simulink model "warp_timer"  (Simulink 7.1)
settings: Solver=ode45  StartTime=0.0  StopTime=1000  RelTol=1e-3
undefined symbols (not defined in the file): gcbh, xlBlockLoadCallback, xlGetSimulinkPeriod
libraries: xbsIndex_r4 x450
(part 3 of 5)

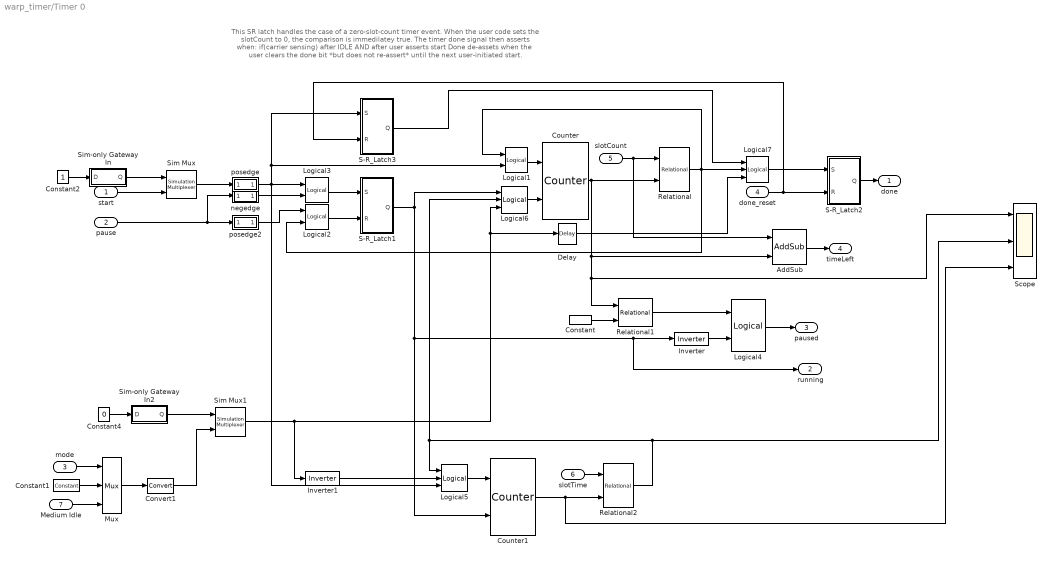
== system warp_timer/Timer 0 ==
  note: This SR latch handles the case of a zero-slot-count
      | timer event. When the user code sets the slotCount to 0,
      | the comparison is immedilatey true. The timer done
      | signal then asserts when:
      | if(carrier sensing) after IDLE AND
      | after user asserts start
      | Done de-assets when the user clears the done bit
      | *but does not re-assert* until the next user-initiated start.
  start : Inport  OutDataType=sfix(16)  OutScaling=2^0
  pause : Inport  Port=2  OutDataType=sfix(16)  OutScaling=2^0
  mode : Inport  Port=3  OutDataType=sfix(16)  OutScaling=2^0
  done_reset : Inport  Port=4  OutDataType=sfix(16)  OutScaling=2^0
  slotCount : Inport  Port=5  OutDataType=sfix(16)  OutScaling=2^0
  slotTime : Inport  Port=6  OutDataType=sfix(16)  OutScaling=2^0
  Medium Idle : Inport  Port=7  OutDataType=sfix(16)  OutScaling=2^0
  AddSub : xbsIndex_r4/AddSub  mode=Subtraction  use_carryin=off  use_carryout=off  en=off  latency=0  precision=User Defined  arith_type=Unsigned  n_bits=32  bin_pt=0  quantization=Truncate  overflow=Wrap  dbl_ovrd=off  use_behavioral_HDL=off  pipelined=off  use_rpm=on  hw_selection=Fabric  block_type=addsub
      settings: xl_area=[16 0 0 32 0 0 0]  block_version=8.2
  Constant : xbsIndex_r4/Constant  arith_type=Unsigned  const=0  n_bits=32  bin_pt=0  explicit_period=off  period=1  equ=P=C  opselect=C  inp2=PCIN>>17  opr=+  inp1=P  carry=CIN  dbl_ovrd=off  block_type=constant
      settings: block_version=10.1.2
  Constant1 : xbsIndex_r4/Constant  arith_type=Unsigned  const=1  n_bits=1  bin_pt=0  explicit_period=off  period=1  equ=P=C  opselect=C  inp2=PCIN>>17  opr=+  inp1=P  carry=CIN  dbl_ovrd=off  block_type=constant
      settings: block_version=8.2
  Constant2 : Constant  OutDataType=sfix(16)  OutScaling=2^0
  Constant4 : Constant  Value=0  OutDataType=sfix(16)  OutScaling=2^0
  Convert1 : xbsIndex_r4/Convert  arith_type=Boolean  n_bits=16  bin_pt=14  quantization=Truncate  overflow=Wrap  latency=0  dbl_ovrd=off  pipeline=off  block_type=convert
      settings: xl_area=[0 0 0 0 0 0 0]  block_version=8.2
  Counter : xbsIndex_r4/Counter  cnt_type=Free Running  cnt_to=Inf  operation=Up  start_count=0  cnt_by_val=1  arith_type=Unsigned  n_bits=32  bin_pt=0  load_pin=off  rst=on  en=on  explicit_period=on  period=1  dbl_ovrd=off  use_behavioral_HDL=off  use_rpm=off  implementation=Fabric  block_type=counter
      settings: xl_area=[17 32 0 32 0 0 0]  block_version=8.2
  Counter1 : xbsIndex_r4/Counter  cnt_type=Free Running  cnt_to=Inf  operation=Up  start_count=0  cnt_by_val=1  arith_type=Unsigned  n_bits=16  bin_pt=0  load_pin=off  rst=on  en=on  explicit_period=on  period=1  dbl_ovrd=off  use_behavioral_HDL=off  use_rpm=off  implementation=Fabric  block_type=counter
      settings: xl_area=[17 32 0 32 0 0 0]  block_version=8.2
  Delay : xbsIndex_r4/Delay  en=off  latency=1  dbl_ovrd=off  reg_retiming=off  block_type=delay
  Inverter : xbsIndex_r4/Inverter  en=off  latency=0  dbl_ovrd=off  block_type=inv
      settings: xl_area=[0 0 0 0 0 0 0]  block_version=10.1.2
  Inverter1 : xbsIndex_r4/Inverter  en=off  latency=0  dbl_ovrd=off  block_type=inv
      settings: xl_area=[0 0 0 0 0 0 0]  block_version=10.1.2
  Logical1 : xbsIndex_r4/Logical  logical_function=OR  inputs=2  en=off  latency=0  precision=Full  arith_type=Unsigned  n_bits=16  bin_pt=0  align_bp=on  dbl_ovrd=off  block_type=logical
      settings: xl_area=[1 0 0 1 0 0 0]  block_version=9.1.01
  Logical2 : xbsIndex_r4/Logical  logical_function=OR  inputs=2  en=off  latency=0  precision=Full  arith_type=Unsigned  n_bits=16  bin_pt=0  align_bp=on  dbl_ovrd=off  block_type=logical
      settings: xl_area=[1 0 0 1 0 0 0]  block_version=9.1.01
  Logical3 : xbsIndex_r4/Logical  logical_function=OR  inputs=2  en=off  latency=0  precision=Full  arith_type=Unsigned  n_bits=16  bin_pt=0  align_bp=on  dbl_ovrd=off  block_type=logical
      settings: xl_area=[1 0 0 1 0 0 0]  block_version=9.1.01
  Logical4 : xbsIndex_r4/Logical  logical_function=AND  inputs=2  en=off  latency=0  precision=Full  arith_type=Unsigned  n_bits=16  bin_pt=0  align_bp=on  dbl_ovrd=off  block_type=logical
      settings: xl_area=[1 0 0 1 0 0 0]  block_version=10.1.2
  Logical5 : xbsIndex_r4/Logical  logical_function=OR  inputs=3  en=off  latency=0  precision=Full  arith_type=Unsigned  n_bits=16  bin_pt=0  align_bp=on  dbl_ovrd=off  block_type=logical
      settings: xl_area=[1 0 0 1 0 0 0]  block_version=8.2
  Logical6 : xbsIndex_r4/Logical  logical_function=AND  inputs=3  en=off  latency=0  precision=Full  arith_type=Unsigned  n_bits=16  bin_pt=0  align_bp=on  dbl_ovrd=off  block_type=logical
      settings: xl_area=[1 0 0 1 0 0 0]  block_version=8.2
  Logical7 : xbsIndex_r4/Logical  logical_function=AND  inputs=3  en=off  latency=0  precision=Full  arith_type=Unsigned  n_bits=16  bin_pt=0  align_bp=on  dbl_ovrd=off  block_type=logical
      settings: xl_area=[1 0 0 1 0 0 0]  block_version=9.1.01
  Mux : xbsIndex_r4/Mux  inputs=2  en=off  latency=0  precision=Full  arith_type=Unsigned  n_bits=16  bin_pt=14  quantization=Truncate  overflow=Wrap  dbl_ovrd=off  block_type=mux
      settings: xl_area=[1 0 0 1 0 0 0]  block_version=8.2
  Relational : xbsIndex_r4/Relational  mode=a<=b  en=off  latency=0  dbl_ovrd=off  block_type=relational
      settings: xl_area=[8 0 0 16 0 0 0]  block_version=8.2
  Relational1 : xbsIndex_r4/Relational  mode=a>b  en=off  latency=0  dbl_ovrd=off  block_type=relational
      settings: xl_area=[16 1 0 32 0 0 0]  block_version=10.1.2
  Relational2 : xbsIndex_r4/Relational  mode=a<=b  en=off  latency=0  dbl_ovrd=off  block_type=relational
      settings: xl_area=[8 0 0 16 0 0 0]  block_version=8.2
  S-R_Latch1 : Subsystem
  S-R_Latch2 : Subsystem
  S-R_Latch3 : Subsystem
  Scope : Scope  NumInputPorts=3
      settings: YMin=-5~-5~-5  YMax=5~5~5
  Sim Mux : xbsIndex_r4/Simulation Multiplexer  sim_sel=1  hw_sel=2  block_type=simmux
      settings: infoedit="Distinguish input subsystems as \"simulation only\" and \"generation only\".  The input specified For Simulation will be used during Simulink simulation.  The input specified For Generation will be used during code generation.  This block will typically be used on the output of a HW Co-Simulation, Black Box, or ModelSim subsystem.<P><P>Hardware Notes: This block costs nothing."  block_version=10.1.3
  Sim Mux1 : xbsIndex_r4/Simulation Multiplexer  sim_sel=1  hw_sel=2  block_type=simmux
      settings: infoedit="Distinguish input subsystems as \"simulation only\" and \"generation only\".  The input specified For Simulation will be used during Simulink simulation.  The input specified For Generation will be used during code generation.  This block will typically be used on the output of a HW Co-Simulation, Black Box, or ModelSim subsystem.<P><P>Hardware Notes: This block costs nothing."  block_version=10.1.3
  Sim-only Gateway In : Subsystem
  Sim-only Gateway In2 : Subsystem
  negedge : Subsystem
  posedge : Subsystem
  posedge2 : Subsystem
  done : Outport  OutDataType=sfix(16)  OutScaling=2^0
  running : Outport  Port=2  OutDataType=sfix(16)  OutScaling=2^0
  paused : Outport  Port=3  OutDataType=sfix(16)  OutScaling=2^0
  timeLeft : Outport  Port=4  OutDataType=sfix(16)  OutScaling=2^0
  wires:
  mode/1 -> Mux/1
  Constant1/1 -> Mux/2
  Medium Idle/1 -> Mux/3
  Mux/1 -> Convert1/1
  Logical4/1 -> paused/1
  start/1 -> Sim Mux/2
  Sim Mux/1 -> posedge/1(In)
  AddSub/1 -> timeLeft/1
  Constant/1 -> Relational1/2
  Relational1/1 -> Logical4/1
  Inverter/1 -> Logical4/2
  S-R_Latch1/1(Q) -> Counter1/2, Inverter/1, running/1, Logical6/1
  slotCount/1 -> AddSub/1, Relational/1
  Counter/1 -> Relational/2, AddSub/2, Relational1/1, Scope/1
  Logical1/1 -> Counter/1
  S-R_Latch2/1(Q) -> done/1
  Relational/1 -> Logical2/2, Logical1/1, Logical7/2
  done_reset/1 -> S-R_Latch2/2(R), S-R_Latch3/2(R)
  posedge/1(Out) -> Logical3/1, Logical5/3, Logical1/2, S-R_Latch3/1(S)
  Logical3/1 -> S-R_Latch1/1(S)
  negedge/1(Out) -> Logical3/2
  pause/1 -> posedge2/1(In), negedge/1(In)
  Sim-only Gateway In/1(Q) -> Sim Mux/1
  slotTime/1 -> Relational2/1
  Counter1/1 -> Relational2/2, Scope/3
  Logical5/1 -> Counter1/1
  Relational2/1 -> Logical5/1, Logical6/2, Scope/2
  Inverter1/1 -> Logical5/2
  Logical6/1 -> Counter/2
  Convert1/1 -> Sim Mux1/2
  Sim Mux1/1 -> Inverter1/1, Logical6/3, Delay/1
  Constant2/1 -> Sim-only Gateway In/1(D)
  posedge2/1(Out) -> Logical2/1
  Logical2/1 -> S-R_Latch1/2(R)
  Constant4/1 -> Sim-only Gateway In2/1(D)
  Sim-only Gateway In2/1(Q) -> Sim Mux1/1
  Logical7/1 -> S-R_Latch2/1(S)
  S-R_Latch3/1(Q) -> Logical7/1
  Delay/1 -> Logical7/3

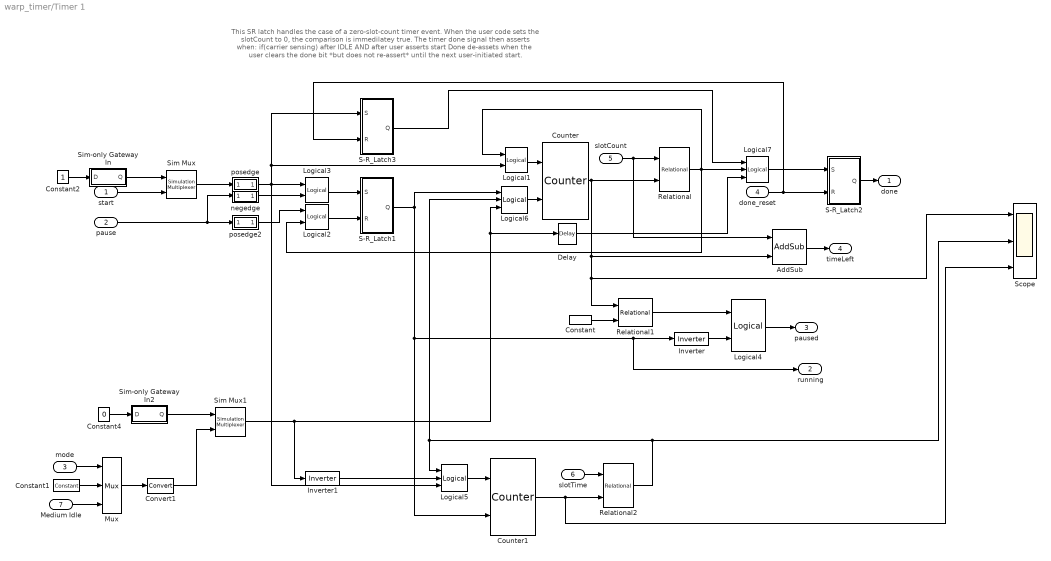
== system warp_timer/Timer 1 ==
  note: This SR latch handles the case of a zero-slot-count
      | timer event. When the user code sets the slotCount to 0,
      | the comparison is immedilatey true. The timer done
      | signal then asserts when:
      | if(carrier sensing) after IDLE AND
      | after user asserts start
      | Done de-assets when the user clears the done bit
      | *but does not re-assert* until the next user-initiated start.
  start : Inport  OutDataType=sfix(16)  OutScaling=2^0
  pause : Inport  Port=2  OutDataType=sfix(16)  OutScaling=2^0
  mode : Inport  Port=3  OutDataType=sfix(16)  OutScaling=2^0
  done_reset : Inport  Port=4  OutDataType=sfix(16)  OutScaling=2^0
  slotCount : Inport  Port=5  OutDataType=sfix(16)  OutScaling=2^0
  slotTime : Inport  Port=6  OutDataType=sfix(16)  OutScaling=2^0
  Medium Idle : Inport  Port=7  OutDataType=sfix(16)  OutScaling=2^0
  AddSub : xbsIndex_r4/AddSub  mode=Subtraction  use_carryin=off  use_carryout=off  en=off  latency=0  precision=User Defined  arith_type=Unsigned  n_bits=32  bin_pt=0  quantization=Truncate  overflow=Wrap  dbl_ovrd=off  use_behavioral_HDL=off  pipelined=off  use_rpm=on  hw_selection=Fabric  block_type=addsub
      settings: xl_area=[16 0 0 32 0 0 0]  block_version=8.2
  Constant : xbsIndex_r4/Constant  arith_type=Unsigned  const=0  n_bits=32  bin_pt=0  explicit_period=off  period=1  equ=P=C  opselect=C  inp2=PCIN>>17  opr=+  inp1=P  carry=CIN  dbl_ovrd=off  block_type=constant
      settings: block_version=10.1.2
  Constant1 : xbsIndex_r4/Constant  arith_type=Unsigned  const=1  n_bits=1  bin_pt=0  explicit_period=off  period=1  equ=P=C  opselect=C  inp2=PCIN>>17  opr=+  inp1=P  carry=CIN  dbl_ovrd=off  block_type=constant
      settings: block_version=8.2
  Constant2 : Constant  OutDataType=sfix(16)  OutScaling=2^0
  Constant4 : Constant  Value=0  OutDataType=sfix(16)  OutScaling=2^0
  Convert1 : xbsIndex_r4/Convert  arith_type=Boolean  n_bits=16  bin_pt=14  quantization=Truncate  overflow=Wrap  latency=0  dbl_ovrd=off  pipeline=off  block_type=convert
      settings: xl_area=[0 0 0 0 0 0 0]  block_version=8.2
  Counter : xbsIndex_r4/Counter  cnt_type=Free Running  cnt_to=Inf  operation=Up  start_count=0  cnt_by_val=1  arith_type=Unsigned  n_bits=32  bin_pt=0  load_pin=off  rst=on  en=on  explicit_period=on  period=1  dbl_ovrd=off  use_behavioral_HDL=off  use_rpm=off  implementation=Fabric  block_type=counter
      settings: xl_area=[17 32 0 32 0 0 0]  block_version=8.2
  Counter1 : xbsIndex_r4/Counter  cnt_type=Free Running  cnt_to=Inf  operation=Up  start_count=0  cnt_by_val=1  arith_type=Unsigned  n_bits=16  bin_pt=0  load_pin=off  rst=on  en=on  explicit_period=on  period=1  dbl_ovrd=off  use_behavioral_HDL=off  use_rpm=off  implementation=Fabric  block_type=counter
      settings: xl_area=[17 32 0 32 0 0 0]  block_version=8.2
  Delay : xbsIndex_r4/Delay  en=off  latency=1  dbl_ovrd=off  reg_retiming=off  block_type=delay
  Inverter : xbsIndex_r4/Inverter  en=off  latency=0  dbl_ovrd=off  block_type=inv
      settings: xl_area=[0 0 0 0 0 0 0]  block_version=10.1.2
  Inverter1 : xbsIndex_r4/Inverter  en=off  latency=0  dbl_ovrd=off  block_type=inv
      settings: xl_area=[0 0 0 0 0 0 0]  block_version=10.1.2
  Logical1 : xbsIndex_r4/Logical  logical_function=OR  inputs=2  en=off  latency=0  precision=Full  arith_type=Unsigned  n_bits=16  bin_pt=0  align_bp=on  dbl_ovrd=off  block_type=logical
      settings: xl_area=[1 0 0 1 0 0 0]  block_version=9.1.01
  Logical2 : xbsIndex_r4/Logical  logical_function=OR  inputs=2  en=off  latency=0  precision=Full  arith_type=Unsigned  n_bits=16  bin_pt=0  align_bp=on  dbl_ovrd=off  block_type=logical
      settings: xl_area=[1 0 0 1 0 0 0]  block_version=9.1.01
  Logical3 : xbsIndex_r4/Logical  logical_function=OR  inputs=2  en=off  latency=0  precision=Full  arith_type=Unsigned  n_bits=16  bin_pt=0  align_bp=on  dbl_ovrd=off  block_type=logical
      settings: xl_area=[1 0 0 1 0 0 0]  block_version=9.1.01
  Logical4 : xbsIndex_r4/Logical  logical_function=AND  inputs=2  en=off  latency=0  precision=Full  arith_type=Unsigned  n_bits=16  bin_pt=0  align_bp=on  dbl_ovrd=off  block_type=logical
      settings: xl_area=[1 0 0 1 0 0 0]  block_version=10.1.2
  Logical5 : xbsIndex_r4/Logical  logical_function=OR  inputs=3  en=off  latency=0  precision=Full  arith_type=Unsigned  n_bits=16  bin_pt=0  align_bp=on  dbl_ovrd=off  block_type=logical
      settings: xl_area=[1 0 0 1 0 0 0]  block_version=8.2
  Logical6 : xbsIndex_r4/Logical  logical_function=AND  inputs=3  en=off  latency=0  precision=Full  arith_type=Unsigned  n_bits=16  bin_pt=0  align_bp=on  dbl_ovrd=off  block_type=logical
      settings: xl_area=[1 0 0 1 0 0 0]  block_version=8.2
  Logical7 : xbsIndex_r4/Logical  logical_function=AND  inputs=3  en=off  latency=0  precision=Full  arith_type=Unsigned  n_bits=16  bin_pt=0  align_bp=on  dbl_ovrd=off  block_type=logical
      settings: xl_area=[1 0 0 1 0 0 0]  block_version=9.1.01
  Mux : xbsIndex_r4/Mux  inputs=2  en=off  latency=0  precision=Full  arith_type=Unsigned  n_bits=16  bin_pt=14  quantization=Truncate  overflow=Wrap  dbl_ovrd=off  block_type=mux
      settings: xl_area=[1 0 0 1 0 0 0]  block_version=8.2
  Relational : xbsIndex_r4/Relational  mode=a<=b  en=off  latency=0  dbl_ovrd=off  block_type=relational
      settings: xl_area=[8 0 0 16 0 0 0]  block_version=8.2
  Relational1 : xbsIndex_r4/Relational  mode=a>b  en=off  latency=0  dbl_ovrd=off  block_type=relational
      settings: xl_area=[16 1 0 32 0 0 0]  block_version=10.1.2
  Relational2 : xbsIndex_r4/Relational  mode=a<=b  en=off  latency=0  dbl_ovrd=off  block_type=relational
      settings: xl_area=[8 0 0 16 0 0 0]  block_version=8.2
  S-R_Latch1 : Subsystem
  S-R_Latch2 : Subsystem
  S-R_Latch3 : Subsystem
  Scope : Scope  NumInputPorts=3
      settings: YMin=-5~-5~-5  YMax=5~5~5
  Sim Mux : xbsIndex_r4/Simulation Multiplexer  sim_sel=1  hw_sel=2  block_type=simmux
      settings: infoedit="Distinguish input subsystems as \"simulation only\" and \"generation only\".  The input specified For Simulation will be used during Simulink simulation.  The input specified For Generation will be used during code generation.  This block will typically be used on the output of a HW Co-Simulation, Black Box, or ModelSim subsystem.<P><P>Hardware Notes: This block costs nothing."  block_version=10.1.3
  Sim Mux1 : xbsIndex_r4/Simulation Multiplexer  sim_sel=1  hw_sel=2  block_type=simmux
      settings: infoedit="Distinguish input subsystems as \"simulation only\" and \"generation only\".  The input specified For Simulation will be used during Simulink simulation.  The input specified For Generation will be used during code generation.  This block will typically be used on the output of a HW Co-Simulation, Black Box, or ModelSim subsystem.<P><P>Hardware Notes: This block costs nothing."  block_version=10.1.3
  Sim-only Gateway In : Subsystem
  Sim-only Gateway In2 : Subsystem
  negedge : Subsystem
  posedge : Subsystem
  posedge2 : Subsystem
  done : Outport  OutDataType=sfix(16)  OutScaling=2^0
  running : Outport  Port=2  OutDataType=sfix(16)  OutScaling=2^0
  paused : Outport  Port=3  OutDataType=sfix(16)  OutScaling=2^0
  timeLeft : Outport  Port=4  OutDataType=sfix(16)  OutScaling=2^0
  wires:
  Delay/1 -> Logical7/3
  S-R_Latch3/1(Q) -> Logical7/1
  Logical7/1 -> S-R_Latch2/1(S)
  Sim-only Gateway In2/1(Q) -> Sim Mux1/1
  Constant4/1 -> Sim-only Gateway In2/1(D)
  Logical2/1 -> S-R_Latch1/2(R)
  posedge2/1(Out) -> Logical2/1
  Constant2/1 -> Sim-only Gateway In/1(D)
  Sim Mux1/1 -> Delay/1, Logical6/3, Inverter1/1
  Convert1/1 -> Sim Mux1/2
  Logical6/1 -> Counter/2
  Inverter1/1 -> Logical5/2
  Relational2/1 -> Scope/2, Logical6/2, Logical5/1
  Logical5/1 -> Counter1/1
  Counter1/1 -> Scope/3, Relational2/2
  slotTime/1 -> Relational2/1
  Sim-only Gateway In/1(Q) -> Sim Mux/1
  pause/1 -> negedge/1(In), posedge2/1(In)
  negedge/1(Out) -> Logical3/2
  Logical3/1 -> S-R_Latch1/1(S)
  posedge/1(Out) -> S-R_Latch3/1(S), Logical1/2, Logical5/3, Logical3/1
  done_reset/1 -> S-R_Latch3/2(R), S-R_Latch2/2(R)
  Relational/1 -> Logical7/2, Logical1/1, Logical2/2
  S-R_Latch2/1(Q) -> done/1
  Logical1/1 -> Counter/1
  Counter/1 -> Scope/1, Relational1/1, AddSub/2, Relational/2
  slotCount/1 -> Relational/1, AddSub/1
  S-R_Latch1/1(Q) -> Logical6/1, running/1, Inverter/1, Counter1/2
  Inverter/1 -> Logical4/2
  Relational1/1 -> Logical4/1
  Constant/1 -> Relational1/2
  AddSub/1 -> timeLeft/1
  Sim Mux/1 -> posedge/1(In)
  start/1 -> Sim Mux/2
  Logical4/1 -> paused/1
  Mux/1 -> Convert1/1
  Medium Idle/1 -> Mux/3
  Constant1/1 -> Mux/2
  mode/1 -> Mux/1

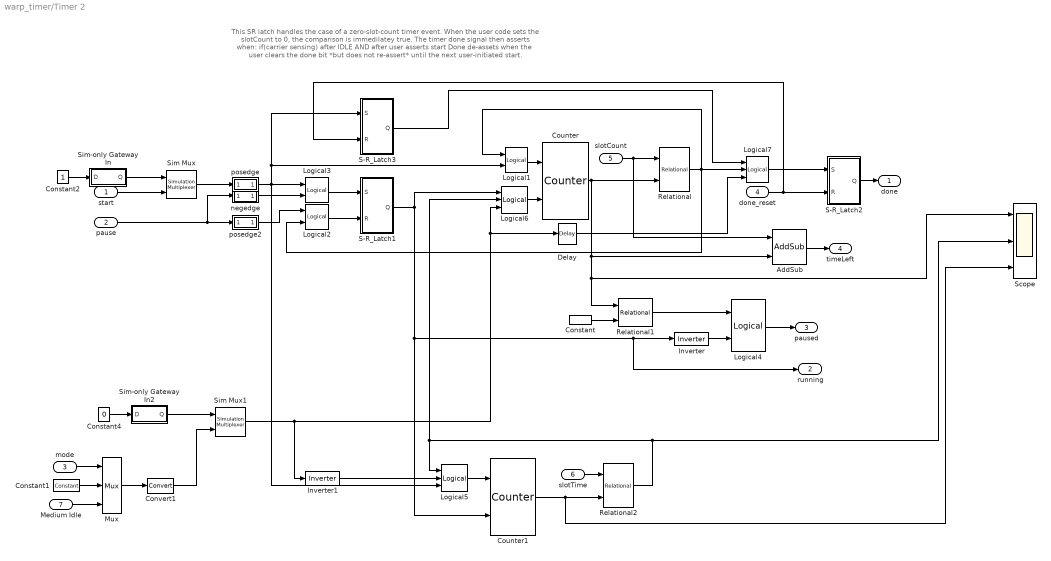
== system warp_timer/Timer 2 ==
  note: This SR latch handles the case of a zero-slot-count
      | timer event. When the user code sets the slotCount to 0,
      | the comparison is immedilatey true. The timer done
      | signal then asserts when:
      | if(carrier sensing) after IDLE AND
      | after user asserts start
      | Done de-assets when the user clears the done bit
      | *but does not re-assert* until the next user-initiated start.
  start : Inport  OutDataType=sfix(16)  OutScaling=2^0
  pause : Inport  Port=2  OutDataType=sfix(16)  OutScaling=2^0
  mode : Inport  Port=3  OutDataType=sfix(16)  OutScaling=2^0
  done_reset : Inport  Port=4  OutDataType=sfix(16)  OutScaling=2^0
  slotCount : Inport  Port=5  OutDataType=sfix(16)  OutScaling=2^0
  slotTime : Inport  Port=6  OutDataType=sfix(16)  OutScaling=2^0
  Medium Idle : Inport  Port=7  OutDataType=sfix(16)  OutScaling=2^0
  AddSub : xbsIndex_r4/AddSub  mode=Subtraction  use_carryin=off  use_carryout=off  en=off  latency=0  precision=User Defined  arith_type=Unsigned  n_bits=32  bin_pt=0  quantization=Truncate  overflow=Wrap  dbl_ovrd=off  use_behavioral_HDL=off  pipelined=off  use_rpm=on  hw_selection=Fabric  block_type=addsub
      settings: xl_area=[16 0 0 32 0 0 0]  block_version=8.2
  Constant : xbsIndex_r4/Constant  arith_type=Unsigned  const=0  n_bits=32  bin_pt=0  explicit_period=off  period=1  equ=P=C  opselect=C  inp2=PCIN>>17  opr=+  inp1=P  carry=CIN  dbl_ovrd=off  block_type=constant
      settings: block_version=10.1.2
  Constant1 : xbsIndex_r4/Constant  arith_type=Unsigned  const=1  n_bits=1  bin_pt=0  explicit_period=off  period=1  equ=P=C  opselect=C  inp2=PCIN>>17  opr=+  inp1=P  carry=CIN  dbl_ovrd=off  block_type=constant
      settings: block_version=8.2
  Constant2 : Constant  OutDataType=sfix(16)  OutScaling=2^0
  Constant4 : Constant  Value=0  OutDataType=sfix(16)  OutScaling=2^0
  Convert1 : xbsIndex_r4/Convert  arith_type=Boolean  n_bits=16  bin_pt=14  quantization=Truncate  overflow=Wrap  latency=0  dbl_ovrd=off  pipeline=off  block_type=convert
      settings: xl_area=[0 0 0 0 0 0 0]  block_version=8.2
  Counter : xbsIndex_r4/Counter  cnt_type=Free Running  cnt_to=Inf  operation=Up  start_count=0  cnt_by_val=1  arith_type=Unsigned  n_bits=32  bin_pt=0  load_pin=off  rst=on  en=on  explicit_period=on  period=1  dbl_ovrd=off  use_behavioral_HDL=off  use_rpm=off  implementation=Fabric  block_type=counter
      settings: xl_area=[17 32 0 32 0 0 0]  block_version=8.2
  Counter1 : xbsIndex_r4/Counter  cnt_type=Free Running  cnt_to=Inf  operation=Up  start_count=0  cnt_by_val=1  arith_type=Unsigned  n_bits=16  bin_pt=0  load_pin=off  rst=on  en=on  explicit_period=on  period=1  dbl_ovrd=off  use_behavioral_HDL=off  use_rpm=off  implementation=Fabric  block_type=counter
      settings: xl_area=[17 32 0 32 0 0 0]  block_version=8.2
  Delay : xbsIndex_r4/Delay  en=off  latency=1  dbl_ovrd=off  reg_retiming=off  block_type=delay
  Inverter : xbsIndex_r4/Inverter  en=off  latency=0  dbl_ovrd=off  block_type=inv
      settings: xl_area=[0 0 0 0 0 0 0]  block_version=10.1.2
  Inverter1 : xbsIndex_r4/Inverter  en=off  latency=0  dbl_ovrd=off  block_type=inv
      settings: xl_area=[0 0 0 0 0 0 0]  block_version=10.1.2
  Logical1 : xbsIndex_r4/Logical  logical_function=OR  inputs=2  en=off  latency=0  precision=Full  arith_type=Unsigned  n_bits=16  bin_pt=0  align_bp=on  dbl_ovrd=off  block_type=logical
      settings: xl_area=[1 0 0 1 0 0 0]  block_version=9.1.01
  Logical2 : xbsIndex_r4/Logical  logical_function=OR  inputs=2  en=off  latency=0  precision=Full  arith_type=Unsigned  n_bits=16  bin_pt=0  align_bp=on  dbl_ovrd=off  block_type=logical
      settings: xl_area=[1 0 0 1 0 0 0]  block_version=9.1.01
  Logical3 : xbsIndex_r4/Logical  logical_function=OR  inputs=2  en=off  latency=0  precision=Full  arith_type=Unsigned  n_bits=16  bin_pt=0  align_bp=on  dbl_ovrd=off  block_type=logical
      settings: xl_area=[1 0 0 1 0 0 0]  block_version=9.1.01
  Logical4 : xbsIndex_r4/Logical  logical_function=AND  inputs=2  en=off  latency=0  precision=Full  arith_type=Unsigned  n_bits=16  bin_pt=0  align_bp=on  dbl_ovrd=off  block_type=logical
      settings: xl_area=[1 0 0 1 0 0 0]  block_version=10.1.2
  Logical5 : xbsIndex_r4/Logical  logical_function=OR  inputs=3  en=off  latency=0  precision=Full  arith_type=Unsigned  n_bits=16  bin_pt=0  align_bp=on  dbl_ovrd=off  block_type=logical
      settings: xl_area=[1 0 0 1 0 0 0]  block_version=8.2
  Logical6 : xbsIndex_r4/Logical  logical_function=AND  inputs=3  en=off  latency=0  precision=Full  arith_type=Unsigned  n_bits=16  bin_pt=0  align_bp=on  dbl_ovrd=off  block_type=logical
      settings: xl_area=[1 0 0 1 0 0 0]  block_version=8.2
  Logical7 : xbsIndex_r4/Logical  logical_function=AND  inputs=3  en=off  latency=0  precision=Full  arith_type=Unsigned  n_bits=16  bin_pt=0  align_bp=on  dbl_ovrd=off  block_type=logical
      settings: xl_area=[1 0 0 1 0 0 0]  block_version=9.1.01
  Mux : xbsIndex_r4/Mux  inputs=2  en=off  latency=0  precision=Full  arith_type=Unsigned  n_bits=16  bin_pt=14  quantization=Truncate  overflow=Wrap  dbl_ovrd=off  block_type=mux
      settings: xl_area=[1 0 0 1 0 0 0]  block_version=8.2
  Relational : xbsIndex_r4/Relational  mode=a<=b  en=off  latency=0  dbl_ovrd=off  block_type=relational
      settings: xl_area=[8 0 0 16 0 0 0]  block_version=8.2
  Relational1 : xbsIndex_r4/Relational  mode=a>b  en=off  latency=0  dbl_ovrd=off  block_type=relational
      settings: xl_area=[16 1 0 32 0 0 0]  block_version=10.1.2
  Relational2 : xbsIndex_r4/Relational  mode=a<=b  en=off  latency=0  dbl_ovrd=off  block_type=relational
      settings: xl_area=[8 0 0 16 0 0 0]  block_version=8.2
  S-R_Latch1 : Subsystem
  S-R_Latch2 : Subsystem
  S-R_Latch3 : Subsystem
  Scope : Scope  NumInputPorts=3
      settings: YMin=-5~-5~-5  YMax=5~5~5
  Sim Mux : xbsIndex_r4/Simulation Multiplexer  sim_sel=1  hw_sel=2  block_type=simmux
      settings: infoedit="Distinguish input subsystems as \"simulation only\" and \"generation only\".  The input specified For Simulation will be used during Simulink simulation.  The input specified For Generation will be used during code generation.  This block will typically be used on the output of a HW Co-Simulation, Black Box, or ModelSim subsystem.<P><P>Hardware Notes: This block costs nothing."  block_version=10.1.3
  Sim Mux1 : xbsIndex_r4/Simulation Multiplexer  sim_sel=1  hw_sel=2  block_type=simmux
      settings: infoedit="Distinguish input subsystems as \"simulation only\" and \"generation only\".  The input specified For Simulation will be used during Simulink simulation.  The input specified For Generation will be used during code generation.  This block will typically be used on the output of a HW Co-Simulation, Black Box, or ModelSim subsystem.<P><P>Hardware Notes: This block costs nothing."  block_version=10.1.3
  Sim-only Gateway In : Subsystem
  Sim-only Gateway In2 : Subsystem
  negedge : Subsystem
  posedge : Subsystem
  posedge2 : Subsystem
  done : Outport  OutDataType=sfix(16)  OutScaling=2^0
  running : Outport  Port=2  OutDataType=sfix(16)  OutScaling=2^0
  paused : Outport  Port=3  OutDataType=sfix(16)  OutScaling=2^0
  timeLeft : Outport  Port=4  OutDataType=sfix(16)  OutScaling=2^0
  wires:
  mode/1 -> Mux/1
  Constant1/1 -> Mux/2
  Medium Idle/1 -> Mux/3
  Mux/1 -> Convert1/1
  Logical4/1 -> paused/1
  start/1 -> Sim Mux/2
  Sim Mux/1 -> posedge/1(In)
  AddSub/1 -> timeLeft/1
  Constant/1 -> Relational1/2
  Relational1/1 -> Logical4/1
  Inverter/1 -> Logical4/2
  S-R_Latch1/1(Q) -> Counter1/2, Inverter/1, running/1, Logical6/1
  slotCount/1 -> AddSub/1, Relational/1
  Counter/1 -> Relational/2, AddSub/2, Relational1/1, Scope/1
  Logical1/1 -> Counter/1
  S-R_Latch2/1(Q) -> done/1
  Relational/1 -> Logical2/2, Logical1/1, Logical7/2
  done_reset/1 -> S-R_Latch2/2(R), S-R_Latch3/2(R)
  posedge/1(Out) -> Logical3/1, Logical5/3, Logical1/2, S-R_Latch3/1(S)
  Logical3/1 -> S-R_Latch1/1(S)
  negedge/1(Out) -> Logical3/2
  pause/1 -> posedge2/1(In), negedge/1(In)
  Sim-only Gateway In/1(Q) -> Sim Mux/1
  slotTime/1 -> Relational2/1
  Counter1/1 -> Relational2/2, Scope/3
  Logical5/1 -> Counter1/1
  Relational2/1 -> Logical5/1, Logical6/2, Scope/2
  Inverter1/1 -> Logical5/2
  Logical6/1 -> Counter/2
  Convert1/1 -> Sim Mux1/2
  Sim Mux1/1 -> Inverter1/1, Logical6/3, Delay/1
  Constant2/1 -> Sim-only Gateway In/1(D)
  posedge2/1(Out) -> Logical2/1
  Logical2/1 -> S-R_Latch1/2(R)
  Constant4/1 -> Sim-only Gateway In2/1(D)
  Sim-only Gateway In2/1(Q) -> Sim Mux1/1
  Logical7/1 -> S-R_Latch2/1(S)
  S-R_Latch3/1(Q) -> Logical7/1
  Delay/1 -> Logical7/3

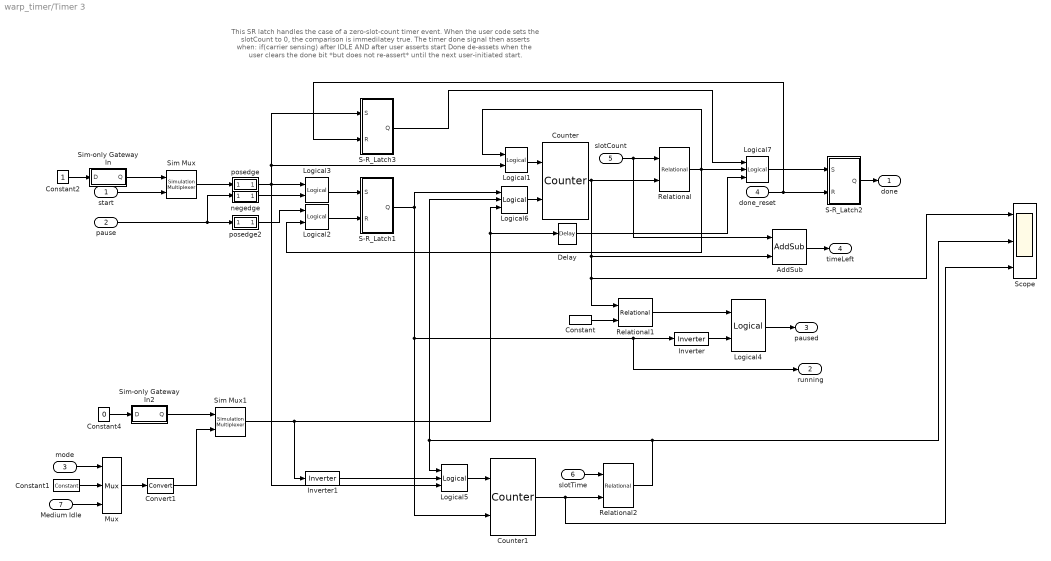
== system warp_timer/Timer 3 ==
  note: This SR latch handles the case of a zero-slot-count
      | timer event. When the user code sets the slotCount to 0,
      | the comparison is immedilatey true. The timer done
      | signal then asserts when:
      | if(carrier sensing) after IDLE AND
      | after user asserts start
      | Done de-assets when the user clears the done bit
      | *but does not re-assert* until the next user-initiated start.
  start : Inport  OutDataType=sfix(16)  OutScaling=2^0
  pause : Inport  Port=2  OutDataType=sfix(16)  OutScaling=2^0
  mode : Inport  Port=3  OutDataType=sfix(16)  OutScaling=2^0
  done_reset : Inport  Port=4  OutDataType=sfix(16)  OutScaling=2^0
  slotCount : Inport  Port=5  OutDataType=sfix(16)  OutScaling=2^0
  slotTime : Inport  Port=6  OutDataType=sfix(16)  OutScaling=2^0
  Medium Idle : Inport  Port=7  OutDataType=sfix(16)  OutScaling=2^0
  AddSub : xbsIndex_r4/AddSub  mode=Subtraction  use_carryin=off  use_carryout=off  en=off  latency=0  precision=User Defined  arith_type=Unsigned  n_bits=32  bin_pt=0  quantization=Truncate  overflow=Wrap  dbl_ovrd=off  use_behavioral_HDL=off  pipelined=off  use_rpm=on  hw_selection=Fabric  block_type=addsub
      settings: xl_area=[16 0 0 32 0 0 0]  block_version=8.2
  Constant : xbsIndex_r4/Constant  arith_type=Unsigned  const=0  n_bits=32  bin_pt=0  explicit_period=off  period=1  equ=P=C  opselect=C  inp2=PCIN>>17  opr=+  inp1=P  carry=CIN  dbl_ovrd=off  block_type=constant
      settings: block_version=10.1.2
  Constant1 : xbsIndex_r4/Constant  arith_type=Unsigned  const=1  n_bits=1  bin_pt=0  explicit_period=off  period=1  equ=P=C  opselect=C  inp2=PCIN>>17  opr=+  inp1=P  carry=CIN  dbl_ovrd=off  block_type=constant
      settings: block_version=8.2
  Constant2 : Constant  OutDataType=sfix(16)  OutScaling=2^0
  Constant4 : Constant  Value=0  OutDataType=sfix(16)  OutScaling=2^0
  Convert1 : xbsIndex_r4/Convert  arith_type=Boolean  n_bits=16  bin_pt=14  quantization=Truncate  overflow=Wrap  latency=0  dbl_ovrd=off  pipeline=off  block_type=convert
      settings: xl_area=[0 0 0 0 0 0 0]  block_version=8.2
  Counter : xbsIndex_r4/Counter  cnt_type=Free Running  cnt_to=Inf  operation=Up  start_count=0  cnt_by_val=1  arith_type=Unsigned  n_bits=32  bin_pt=0  load_pin=off  rst=on  en=on  explicit_period=on  period=1  dbl_ovrd=off  use_behavioral_HDL=off  use_rpm=off  implementation=Fabric  block_type=counter
      settings: xl_area=[17 32 0 32 0 0 0]  block_version=8.2
  Counter1 : xbsIndex_r4/Counter  cnt_type=Free Running  cnt_to=Inf  operation=Up  start_count=0  cnt_by_val=1  arith_type=Unsigned  n_bits=16  bin_pt=0  load_pin=off  rst=on  en=on  explicit_period=on  period=1  dbl_ovrd=off  use_behavioral_HDL=off  use_rpm=off  implementation=Fabric  block_type=counter
      settings: xl_area=[17 32 0 32 0 0 0]  block_version=8.2
  Delay : xbsIndex_r4/Delay  en=off  latency=1  dbl_ovrd=off  reg_retiming=off  block_type=delay
  Inverter : xbsIndex_r4/Inverter  en=off  latency=0  dbl_ovrd=off  block_type=inv
      settings: xl_area=[0 0 0 0 0 0 0]  block_version=10.1.2
  Inverter1 : xbsIndex_r4/Inverter  en=off  latency=0  dbl_ovrd=off  block_type=inv
      settings: xl_area=[0 0 0 0 0 0 0]  block_version=10.1.2
  Logical1 : xbsIndex_r4/Logical  logical_function=OR  inputs=2  en=off  latency=0  precision=Full  arith_type=Unsigned  n_bits=16  bin_pt=0  align_bp=on  dbl_ovrd=off  block_type=logical
      settings: xl_area=[1 0 0 1 0 0 0]  block_version=9.1.01
  Logical2 : xbsIndex_r4/Logical  logical_function=OR  inputs=2  en=off  latency=0  precision=Full  arith_type=Unsigned  n_bits=16  bin_pt=0  align_bp=on  dbl_ovrd=off  block_type=logical
      settings: xl_area=[1 0 0 1 0 0 0]  block_version=9.1.01
  Logical3 : xbsIndex_r4/Logical  logical_function=OR  inputs=2  en=off  latency=0  precision=Full  arith_type=Unsigned  n_bits=16  bin_pt=0  align_bp=on  dbl_ovrd=off  block_type=logical
      settings: xl_area=[1 0 0 1 0 0 0]  block_version=9.1.01
  Logical4 : xbsIndex_r4/Logical  logical_function=AND  inputs=2  en=off  latency=0  precision=Full  arith_type=Unsigned  n_bits=16  bin_pt=0  align_bp=on  dbl_ovrd=off  block_type=logical
      settings: xl_area=[1 0 0 1 0 0 0]  block_version=10.1.2
  Logical5 : xbsIndex_r4/Logical  logical_function=OR  inputs=3  en=off  latency=0  precision=Full  arith_type=Unsigned  n_bits=16  bin_pt=0  align_bp=on  dbl_ovrd=off  block_type=logical
      settings: xl_area=[1 0 0 1 0 0 0]  block_version=8.2
  Logical6 : xbsIndex_r4/Logical  logical_function=AND  inputs=3  en=off  latency=0  precision=Full  arith_type=Unsigned  n_bits=16  bin_pt=0  align_bp=on  dbl_ovrd=off  block_type=logical
      settings: xl_area=[1 0 0 1 0 0 0]  block_version=8.2
  Logical7 : xbsIndex_r4/Logical  logical_function=AND  inputs=3  en=off  latency=0  precision=Full  arith_type=Unsigned  n_bits=16  bin_pt=0  align_bp=on  dbl_ovrd=off  block_type=logical
      settings: xl_area=[1 0 0 1 0 0 0]  block_version=9.1.01
  Mux : xbsIndex_r4/Mux  inputs=2  en=off  latency=0  precision=Full  arith_type=Unsigned  n_bits=16  bin_pt=14  quantization=Truncate  overflow=Wrap  dbl_ovrd=off  block_type=mux
      settings: xl_area=[1 0 0 1 0 0 0]  block_version=8.2
  Relational : xbsIndex_r4/Relational  mode=a<=b  en=off  latency=0  dbl_ovrd=off  block_type=relational
      settings: xl_area=[8 0 0 16 0 0 0]  block_version=8.2
  Relational1 : xbsIndex_r4/Relational  mode=a>b  en=off  latency=0  dbl_ovrd=off  block_type=relational
      settings: xl_area=[16 1 0 32 0 0 0]  block_version=10.1.2
  Relational2 : xbsIndex_r4/Relational  mode=a<=b  en=off  latency=0  dbl_ovrd=off  block_type=relational
      settings: xl_area=[8 0 0 16 0 0 0]  block_version=8.2
  S-R_Latch1 : Subsystem
  S-R_Latch2 : Subsystem
  S-R_Latch3 : Subsystem
  Scope : Scope  NumInputPorts=3
      settings: YMin=-5~-5~-5  YMax=5~5~5
  Sim Mux : xbsIndex_r4/Simulation Multiplexer  sim_sel=1  hw_sel=2  block_type=simmux
      settings: infoedit="Distinguish input subsystems as \"simulation only\" and \"generation only\".  The input specified For Simulation will be used during Simulink simulation.  The input specified For Generation will be used during code generation.  This block will typically be used on the output of a HW Co-Simulation, Black Box, or ModelSim subsystem.<P><P>Hardware Notes: This block costs nothing."  block_version=10.1.3
  Sim Mux1 : xbsIndex_r4/Simulation Multiplexer  sim_sel=1  hw_sel=2  block_type=simmux
      settings: infoedit="Distinguish input subsystems as \"simulation only\" and \"generation only\".  The input specified For Simulation will be used during Simulink simulation.  The input specified For Generation will be used during code generation.  This block will typically be used on the output of a HW Co-Simulation, Black Box, or ModelSim subsystem.<P><P>Hardware Notes: This block costs nothing."  block_version=10.1.3
  Sim-only Gateway In : Subsystem
  Sim-only Gateway In2 : Subsystem
  negedge : Subsystem
  posedge : Subsystem
  posedge2 : Subsystem
  done : Outport  OutDataType=sfix(16)  OutScaling=2^0
  running : Outport  Port=2  OutDataType=sfix(16)  OutScaling=2^0
  paused : Outport  Port=3  OutDataType=sfix(16)  OutScaling=2^0
  timeLeft : Outport  Port=4  OutDataType=sfix(16)  OutScaling=2^0
  wires:
  Delay/1 -> Logical7/3
  S-R_Latch3/1(Q) -> Logical7/1
  Logical7/1 -> S-R_Latch2/1(S)
  Sim-only Gateway In2/1(Q) -> Sim Mux1/1
  Constant4/1 -> Sim-only Gateway In2/1(D)
  Logical2/1 -> S-R_Latch1/2(R)
  posedge2/1(Out) -> Logical2/1
  Constant2/1 -> Sim-only Gateway In/1(D)
  Sim Mux1/1 -> Delay/1, Logical6/3, Inverter1/1
  Convert1/1 -> Sim Mux1/2
  Logical6/1 -> Counter/2
  Inverter1/1 -> Logical5/2
  Relational2/1 -> Scope/2, Logical6/2, Logical5/1
  Logical5/1 -> Counter1/1
  Counter1/1 -> Scope/3, Relational2/2
  slotTime/1 -> Relational2/1
  Sim-only Gateway In/1(Q) -> Sim Mux/1
  pause/1 -> negedge/1(In), posedge2/1(In)
  negedge/1(Out) -> Logical3/2
  Logical3/1 -> S-R_Latch1/1(S)
  posedge/1(Out) -> S-R_Latch3/1(S), Logical1/2, Logical5/3, Logical3/1
  done_reset/1 -> S-R_Latch3/2(R), S-R_Latch2/2(R)
  Relational/1 -> Logical7/2, Logical1/1, Logical2/2
  S-R_Latch2/1(Q) -> done/1
  Logical1/1 -> Counter/1
  Counter/1 -> Scope/1, Relational1/1, AddSub/2, Relational/2
  slotCount/1 -> Relational/1, AddSub/1
  S-R_Latch1/1(Q) -> Logical6/1, running/1, Inverter/1, Counter1/2
  Inverter/1 -> Logical4/2
  Relational1/1 -> Logical4/1
  Constant/1 -> Relational1/2
  AddSub/1 -> timeLeft/1
  Sim Mux/1 -> posedge/1(In)
  start/1 -> Sim Mux/2
  Logical4/1 -> paused/1
  Mux/1 -> Convert1/1
  Medium Idle/1 -> Mux/3
  Constant1/1 -> Mux/2
  mode/1 -> Mux/1

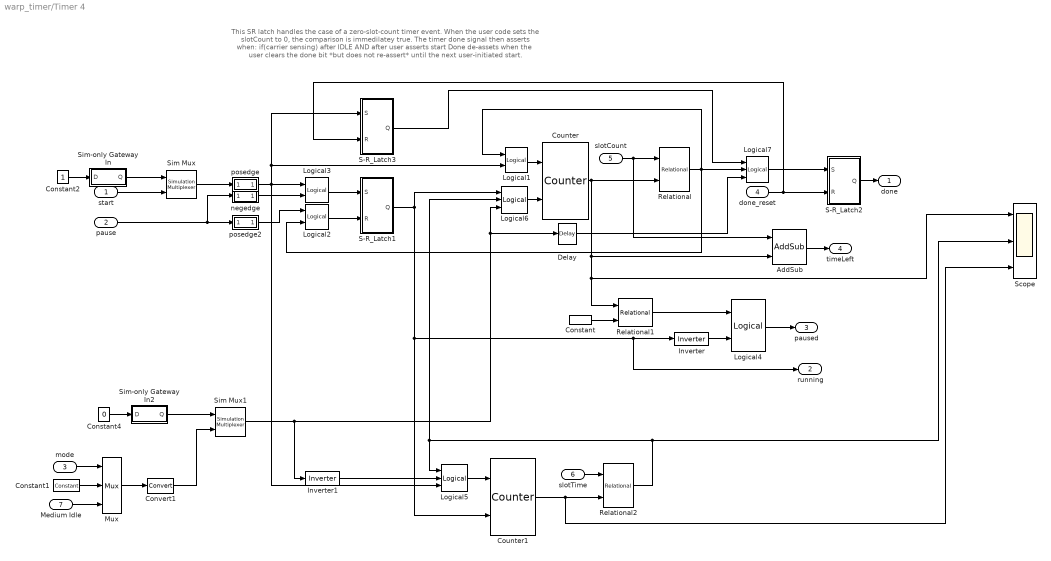
== system warp_timer/Timer 4 ==
  note: This SR latch handles the case of a zero-slot-count
      | timer event. When the user code sets the slotCount to 0,
      | the comparison is immedilatey true. The timer done
      | signal then asserts when:
      | if(carrier sensing) after IDLE AND
      | after user asserts start
      | Done de-assets when the user clears the done bit
      | *but does not re-assert* until the next user-initiated start.
  start : Inport  OutDataType=sfix(16)  OutScaling=2^0
  pause : Inport  Port=2  OutDataType=sfix(16)  OutScaling=2^0
  mode : Inport  Port=3  OutDataType=sfix(16)  OutScaling=2^0
  done_reset : Inport  Port=4  OutDataType=sfix(16)  OutScaling=2^0
  slotCount : Inport  Port=5  OutDataType=sfix(16)  OutScaling=2^0
  slotTime : Inport  Port=6  OutDataType=sfix(16)  OutScaling=2^0
  Medium Idle : Inport  Port=7  OutDataType=sfix(16)  OutScaling=2^0
  AddSub : xbsIndex_r4/AddSub  mode=Subtraction  use_carryin=off  use_carryout=off  en=off  latency=0  precision=User Defined  arith_type=Unsigned  n_bits=32  bin_pt=0  quantization=Truncate  overflow=Wrap  dbl_ovrd=off  use_behavioral_HDL=off  pipelined=off  use_rpm=on  hw_selection=Fabric  block_type=addsub
      settings: xl_area=[16 0 0 32 0 0 0]  block_version=8.2
  Constant : xbsIndex_r4/Constant  arith_type=Unsigned  const=0  n_bits=32  bin_pt=0  explicit_period=off  period=1  equ=P=C  opselect=C  inp2=PCIN>>17  opr=+  inp1=P  carry=CIN  dbl_ovrd=off  block_type=constant
      settings: block_version=10.1.2
  Constant1 : xbsIndex_r4/Constant  arith_type=Unsigned  const=1  n_bits=1  bin_pt=0  explicit_period=off  period=1  equ=P=C  opselect=C  inp2=PCIN>>17  opr=+  inp1=P  carry=CIN  dbl_ovrd=off  block_type=constant
      settings: block_version=8.2
  Constant2 : Constant  OutDataType=sfix(16)  OutScaling=2^0
  Constant4 : Constant  Value=0  OutDataType=sfix(16)  OutScaling=2^0
  Convert1 : xbsIndex_r4/Convert  arith_type=Boolean  n_bits=16  bin_pt=14  quantization=Truncate  overflow=Wrap  latency=0  dbl_ovrd=off  pipeline=off  block_type=convert
      settings: xl_area=[0 0 0 0 0 0 0]  block_version=8.2
  Counter : xbsIndex_r4/Counter  cnt_type=Free Running  cnt_to=Inf  operation=Up  start_count=0  cnt_by_val=1  arith_type=Unsigned  n_bits=32  bin_pt=0  load_pin=off  rst=on  en=on  explicit_period=on  period=1  dbl_ovrd=off  use_behavioral_HDL=off  use_rpm=off  implementation=Fabric  block_type=counter
      settings: xl_area=[17 32 0 32 0 0 0]  block_version=8.2
  Counter1 : xbsIndex_r4/Counter  cnt_type=Free Running  cnt_to=Inf  operation=Up  start_count=0  cnt_by_val=1  arith_type=Unsigned  n_bits=16  bin_pt=0  load_pin=off  rst=on  en=on  explicit_period=on  period=1  dbl_ovrd=off  use_behavioral_HDL=off  use_rpm=off  implementation=Fabric  block_type=counter
      settings: xl_area=[17 32 0 32 0 0 0]  block_version=8.2
  Delay : xbsIndex_r4/Delay  en=off  latency=1  dbl_ovrd=off  reg_retiming=off  block_type=delay
  Inverter : xbsIndex_r4/Inverter  en=off  latency=0  dbl_ovrd=off  block_type=inv
      settings: xl_area=[0 0 0 0 0 0 0]  block_version=10.1.2
  Inverter1 : xbsIndex_r4/Inverter  en=off  latency=0  dbl_ovrd=off  block_type=inv
      settings: xl_area=[0 0 0 0 0 0 0]  block_version=10.1.2
  Logical1 : xbsIndex_r4/Logical  logical_function=OR  inputs=2  en=off  latency=0  precision=Full  arith_type=Unsigned  n_bits=16  bin_pt=0  align_bp=on  dbl_ovrd=off  block_type=logical
      settings: xl_area=[1 0 0 1 0 0 0]  block_version=9.1.01
  Logical2 : xbsIndex_r4/Logical  logical_function=OR  inputs=2  en=off  latency=0  precision=Full  arith_type=Unsigned  n_bits=16  bin_pt=0  align_bp=on  dbl_ovrd=off  block_type=logical
      settings: xl_area=[1 0 0 1 0 0 0]  block_version=9.1.01
  Logical3 : xbsIndex_r4/Logical  logical_function=OR  inputs=2  en=off  latency=0  precision=Full  arith_type=Unsigned  n_bits=16  bin_pt=0  align_bp=on  dbl_ovrd=off  block_type=logical
      settings: xl_area=[1 0 0 1 0 0 0]  block_version=9.1.01
  Logical4 : xbsIndex_r4/Logical  logical_function=AND  inputs=2  en=off  latency=0  precision=Full  arith_type=Unsigned  n_bits=16  bin_pt=0  align_bp=on  dbl_ovrd=off  block_type=logical
      settings: xl_area=[1 0 0 1 0 0 0]  block_version=10.1.2
  Logical5 : xbsIndex_r4/Logical  logical_function=OR  inputs=3  en=off  latency=0  precision=Full  arith_type=Unsigned  n_bits=16  bin_pt=0  align_bp=on  dbl_ovrd=off  block_type=logical
      settings: xl_area=[1 0 0 1 0 0 0]  block_version=8.2
  Logical6 : xbsIndex_r4/Logical  logical_function=AND  inputs=3  en=off  latency=0  precision=Full  arith_type=Unsigned  n_bits=16  bin_pt=0  align_bp=on  dbl_ovrd=off  block_type=logical
      settings: xl_area=[1 0 0 1 0 0 0]  block_version=8.2
  Logical7 : xbsIndex_r4/Logical  logical_function=AND  inputs=3  en=off  latency=0  precision=Full  arith_type=Unsigned  n_bits=16  bin_pt=0  align_bp=on  dbl_ovrd=off  block_type=logical
      settings: xl_area=[1 0 0 1 0 0 0]  block_version=9.1.01
  Mux : xbsIndex_r4/Mux  inputs=2  en=off  latency=0  precision=Full  arith_type=Unsigned  n_bits=16  bin_pt=14  quantization=Truncate  overflow=Wrap  dbl_ovrd=off  block_type=mux
      settings: xl_area=[1 0 0 1 0 0 0]  block_version=8.2
  Relational : xbsIndex_r4/Relational  mode=a<=b  en=off  latency=0  dbl_ovrd=off  block_type=relational
      settings: xl_area=[8 0 0 16 0 0 0]  block_version=8.2
  Relational1 : xbsIndex_r4/Relational  mode=a>b  en=off  latency=0  dbl_ovrd=off  block_type=relational
      settings: xl_area=[16 1 0 32 0 0 0]  block_version=10.1.2
  Relational2 : xbsIndex_r4/Relational  mode=a<=b  en=off  latency=0  dbl_ovrd=off  block_type=relational
      settings: xl_area=[8 0 0 16 0 0 0]  block_version=8.2
  S-R_Latch1 : Subsystem
  S-R_Latch2 : Subsystem
  S-R_Latch3 : Subsystem
  Scope : Scope  NumInputPorts=3
      settings: YMin=-5~-5~-5  YMax=5~5~5
  Sim Mux : xbsIndex_r4/Simulation Multiplexer  sim_sel=1  hw_sel=2  block_type=simmux
      settings: infoedit="Distinguish input subsystems as \"simulation only\" and \"generation only\".  The input specified For Simulation will be used during Simulink simulation.  The input specified For Generation will be used during code generation.  This block will typically be used on the output of a HW Co-Simulation, Black Box, or ModelSim subsystem.<P><P>Hardware Notes: This block costs nothing."  block_version=10.1.3
  Sim Mux1 : xbsIndex_r4/Simulation Multiplexer  sim_sel=1  hw_sel=2  block_type=simmux
      settings: infoedit="Distinguish input subsystems as \"simulation only\" and \"generation only\".  The input specified For Simulation will be used during Simulink simulation.  The input specified For Generation will be used during code generation.  This block will typically be used on the output of a HW Co-Simulation, Black Box, or ModelSim subsystem.<P><P>Hardware Notes: This block costs nothing."  block_version=10.1.3
  Sim-only Gateway In : Subsystem
  Sim-only Gateway In2 : Subsystem
  negedge : Subsystem
  posedge : Subsystem
  posedge2 : Subsystem
  done : Outport  OutDataType=sfix(16)  OutScaling=2^0
  running : Outport  Port=2  OutDataType=sfix(16)  OutScaling=2^0
  paused : Outport  Port=3  OutDataType=sfix(16)  OutScaling=2^0
  timeLeft : Outport  Port=4  OutDataType=sfix(16)  OutScaling=2^0
  wires:
  mode/1 -> Mux/1
  Constant1/1 -> Mux/2
  Medium Idle/1 -> Mux/3
  Mux/1 -> Convert1/1
  Logical4/1 -> paused/1
  start/1 -> Sim Mux/2
  Sim Mux/1 -> posedge/1(In)
  AddSub/1 -> timeLeft/1
  Constant/1 -> Relational1/2
  Relational1/1 -> Logical4/1
  Inverter/1 -> Logical4/2
  S-R_Latch1/1(Q) -> Counter1/2, Inverter/1, running/1, Logical6/1
  slotCount/1 -> AddSub/1, Relational/1
  Counter/1 -> Relational/2, AddSub/2, Relational1/1, Scope/1
  Logical1/1 -> Counter/1
  S-R_Latch2/1(Q) -> done/1
  Relational/1 -> Logical2/2, Logical1/1, Logical7/2
  done_reset/1 -> S-R_Latch2/2(R), S-R_Latch3/2(R)
  posedge/1(Out) -> Logical3/1, Logical5/3, Logical1/2, S-R_Latch3/1(S)
  Logical3/1 -> S-R_Latch1/1(S)
  negedge/1(Out) -> Logical3/2
  pause/1 -> posedge2/1(In), negedge/1(In)
  Sim-only Gateway In/1(Q) -> Sim Mux/1
  slotTime/1 -> Relational2/1
  Counter1/1 -> Relational2/2, Scope/3
  Logical5/1 -> Counter1/1
  Relational2/1 -> Logical5/1, Logical6/2, Scope/2
  Inverter1/1 -> Logical5/2
  Logical6/1 -> Counter/2
  Convert1/1 -> Sim Mux1/2
  Sim Mux1/1 -> Inverter1/1, Logical6/3, Delay/1
  Constant2/1 -> Sim-only Gateway In/1(D)
  posedge2/1(Out) -> Logical2/1
  Logical2/1 -> S-R_Latch1/2(R)
  Constant4/1 -> Sim-only Gateway In2/1(D)
  Sim-only Gateway In2/1(Q) -> Sim Mux1/1
  Logical7/1 -> S-R_Latch2/1(S)
  S-R_Latch3/1(Q) -> Logical7/1
  Delay/1 -> Logical7/3
